simulink model "parte1_eje16_controlAA"  (Simulink 8.1)
settings: Solver=ode45  SolverMode=SingleTasking  StartTime=0.0  StopTime=10.0  RelTol=1e-3
settings Model: Creator=cjuar  LastModifiedBy=cjuar  CovMetricSettings=dwe  CovHtmlReporting=off  covSaveCumulativeToWorkspaceVar=off  CovSaveSingleToWorkspaceVar=off  CovExternalEMLEnable=on
settings DataIOCC: LimitDataPoints=off  SaveFormat=StructureWithTime  SignalLoggingSaveFormat=Dataset
settings OptimizationCC: ExpressionDepthLimit=128
settings DebuggingCC: UnderspecifiedInitializationDetection=Simplified  MergeDetectMultiDrivingBlocksExec=error  SolverPrmCheckMsg=none  FcnCallInpInsideContextMsg=EnableAllAsError  FrameProcessingCompatibilityMsg=error  StateNameClashWarn=none  SFUnexpectedBacktrackingDiag=error  SFNoUnconditionalDefaultTransitionDiag=error
settings HardwareCC: ProdBitPerPointer=64  ProdLargestAtomicFloat=Float  ProdIntDivRoundTo=Zero  ProdEndianess=LittleEndian  ProdHWDeviceType=Specified
settings ModelReferenceCC: PropagateSignalLabelsOutOfModel=on
settings GRTTargetCC: CodeReplacementLibrary=C99 (ISO)  GeneratePreprocessorConditionals=Use local settings  CombineOutputUpdateFcns=on  GRTInterface=off

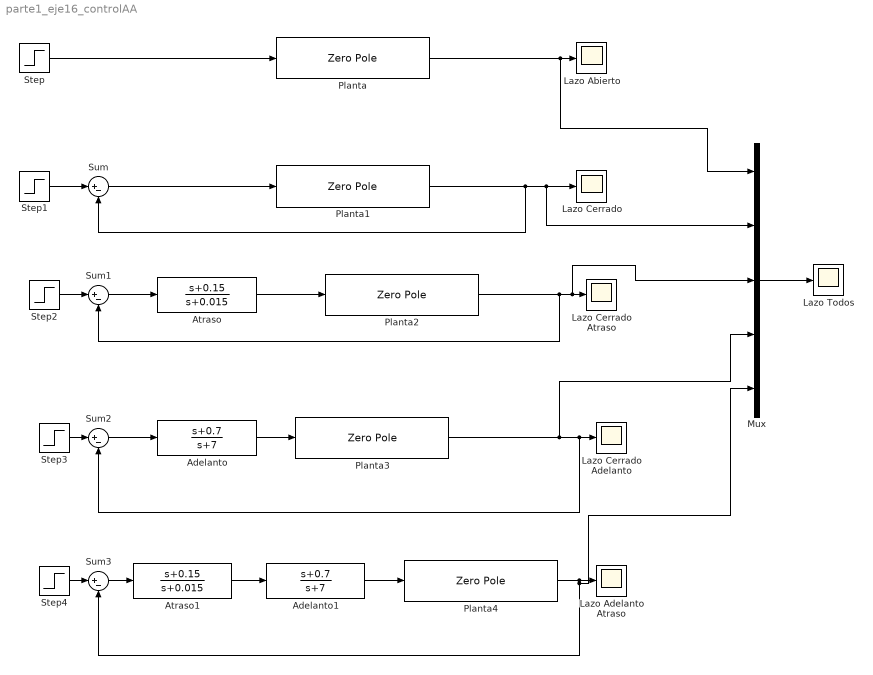
== system parte1_eje16_controlAA ==
  Adelanto : TransferFcn  Numerator=[1 0.7]  Denominator=[1 7]
  Adelanto1 : TransferFcn  Numerator=[1 0.7]  Denominator=[1 7]
  Atraso : TransferFcn  Numerator=[1 0.15]  Denominator=[1 0.015]
  Atraso1 : TransferFcn  Numerator=[1 0.15]  Denominator=[1 0.015]
  Lazo Abierto : Scope
      settings: TimeRange=auto  MaxDataPoints=5000  SaveToWorkspace=off  SaveName=ScopeData  YMin=-9.37531  YMax=84.37778  SampleTime=-1
  Lazo Adelanto Atraso : Scope
      settings: TimeRange=auto  MaxDataPoints=5000  SaveToWorkspace=off  SaveName=ScopeData4  YMin=-0.14583  YMax=1.31246  SampleTime=-1
  Lazo Cerrado : Scope
      settings: TimeRange=auto  MaxDataPoints=5000  SaveToWorkspace=off  YMin=-33.74869  YMax=22.85185  SampleTime=-1
  Lazo Cerrado Adelanto : Scope
      settings: TimeRange=auto  MaxDataPoints=5000  SaveToWorkspace=off  SaveName=ScopeData3  YMin=-0.13101  YMax=1.17912  SampleTime=-1
  Lazo Cerrado Atraso : Scope
      settings: TimeRange=auto  MaxDataPoints=5000  SaveToWorkspace=off  SaveName=ScopeData2  YMin=-55.29579  YMax=34.3255  SampleTime=-1
  Lazo Todos : Scope
      settings: TimeRange=auto  ShowLegends=on  MaxDataPoints=5000  SaveToWorkspace=off  SaveName=ScopeData5  YMin=0.52804  YMax=1.6736  SampleTime=-1
  Mux : Mux  Inputs=5
  Planta{,1..4} (5 alike) : ZeroPole  Zeros=[]  Poles=[0 -1 -2]  Gain=[20]
  Step{,1..4} (5 alike) : Step  SampleTime=0
  Sum{,1..3} (4 alike) : Sum  Inputs=|+-
  wires:
  Step/1 -> Planta/1
  Planta/1 -> Mux/1, Lazo Abierto/1
  Planta1/1 -> Sum/2, Mux/2, Lazo Cerrado/1
  Step1/1 -> Sum/1
  Planta2/1 -> Sum1/2, Mux/3, Lazo Cerrado Atraso/1
  Planta3/1 -> Mux/4, Sum2/2, Lazo Cerrado Adelanto/1
  Sum/1 -> Planta1/1
  Atraso/1 -> Planta2/1
  Adelanto/1 -> Planta3/1
  Step2/1 -> Sum1/1
  Sum1/1 -> Atraso/1
  Step3/1 -> Sum2/1
  Sum2/1 -> Adelanto/1
  Sum3/1 -> Atraso1/1
  Planta4/1 -> Mux/5, Sum3/2, Lazo Adelanto Atraso/1
  Atraso1/1 -> Adelanto1/1
  Step4/1 -> Sum3/1
  Adelanto1/1 -> Planta4/1
  Mux/1 -> Lazo Todos/1
